simulink model "PV_MEV"  (R2025a)
settings: Solver=VariableStepAuto  StartTime=0.0  StopTime=10.0  RelTol=1e-3
InitFcn:
  | init_paras
values from neighbouring files (symbols this model uses):
  C_PFC = 2600e-6    (= 0.0026)    [init_paras.m]
  chg_ctrl_par = [Icc Vcv V_hys T_hys Kp_v_chg Ki_v_chg Kp_i_chg Ki_i_chg Ts_chg D_max_chg t_chg_on k_chg]    [init_paras.m]
  chg_ev = [0 Icc]    [init_paras.m]
  chg_par = [L_chg Voc Rint Ts_chg I_SIGN t_chg_on]    [init_paras.m]
  D = struct('X', {}, 'ti', {}, 'ia', {}, 'tc', {}, 'irms', {}, 'thd', {}, 'trip', {}, 'ttrip', {})    [make_waveform_figs.m]    (also in run_benchmark.m = get_sig('D'))
  det_ema_alpha = 0.1    [init_paras.m]
  det_force = 0    [init_paras.m]
  det_hyst = 0.6    [init_paras.m]
  det_persist = 2    [init_paras.m]
  det_src = 0    [init_paras.m]
  det_t_arm = 0.58    [init_paras.m]
  det_thr = [0.5 0.5 0.5 0.5 0.5]    [init_paras.m]
  det_variant_onehot = double(det_vlist == VARIANT_NAME)    [init_paras.m]
  ENABLE_HIL = 0    [init_paras.m]
  ENABLE_HIL_DET = 0    [init_paras.m]
  ENABLE_HIL_EST = 0    [init_paras.m]
  estimation_src = cfg_row.estimation_src    [init_paras.m]
  Fnom = 50    [init_paras.m]
  Fr_I = Fnom*2    (= 100)    [init_paras.m]
  grid_df = 0    [init_paras.m]
  grid_h5 = 0    [init_paras.m]
  grid_h7 = 0    [init_paras.m]
  grid_var_t0 = 0.7    [init_paras.m]
  hgq_fusion_alpha = [0.6704476522845647 0.7221651725151749 0.6446423751787858 0.41926421682656173]    [init_paras.m]
  hgq_min_ratio = single(0)    [init_paras.m]
  inj_channel = INJ.channel    [init_paras.m]
  inj_dwell = INJ.dwell    [init_paras.m]
  inj_shape = INJ.shape    [init_paras.m]
  inj_t_on = INJ.t_on    [init_paras.m]
  Ki_V = 80    [init_paras.m]
  Kp_I = 0.06    [init_paras.m]
  Kp_V = 0.25    [init_paras.m]
  Kr_I = 2.5    [init_paras.m]
  L_PFC = 600e-6    (= 0.0006)    [init_paras.m]
  Limit_V = 100    [init_paras.m]
  mit_t_ramp = 0.06    [init_paras.m]
  mitigation_mask = 0    [init_paras.m]
  mm_10cycle_points = mm_points_per_cycle * 10    (= 800)    [init_paras.m]
  mm_fund_freq = 50    [init_paras.m]
  mm_points_per_cycle = 80    [init_paras.m]
  R_bleed = 100e3    (= 100000)    [init_paras.m]
  R_pre = Ro*2    (= 44.44)    [init_paras.m]
  res_par = double(RES.par(:)'); end    [init_paras.m]
  RL_PFC = 20e-3    (= 0.02)    [init_paras.m]
  Ro = 22.22    [init_paras.m]
  t_pre_off = 0.30    (= 0.3)    [init_paras.m]
  Ts_chg = 10e-6    (= 1e-05)    [init_paras.m]
  Ts_Control = 1/Fc    [init_paras.m]
  Ts_Power = 50e-9    (= 5e-08)    [init_paras.m]    (also in run_benchmark.m = evalin('base','Ts_Power'))
  use_d_predict = cfg_row.use_d_predict    [init_paras.m]
  use_detector = 0    [init_paras.m]
  use_harmonic = cfg_row.use_harmonic    [init_paras.m]
  use_p_predict = cfg_row.use_p_predict    [init_paras.m]
  Vnom_ac = 240    [init_paras.m]
  vref_ev = [0 0]    [init_paras.m]
undefined symbols (not defined in the file or in its folder): D1, Delta, DiscIntNeverNeededParam
libraries: spsSeriesRLCBranchLib x17, spsMeanLib x16, MyLibrary x12, spsCurrentMeasurementLib x9, spsFourierLib x8, spsTHDLib x8, spsVoltageMeasurementLib x8, spsDiodeLib x7, simulink x7, pycoexlib x5, instrumentlib x4, spsPWMGeneratorDCDCLib x4
(part 4 of 7)

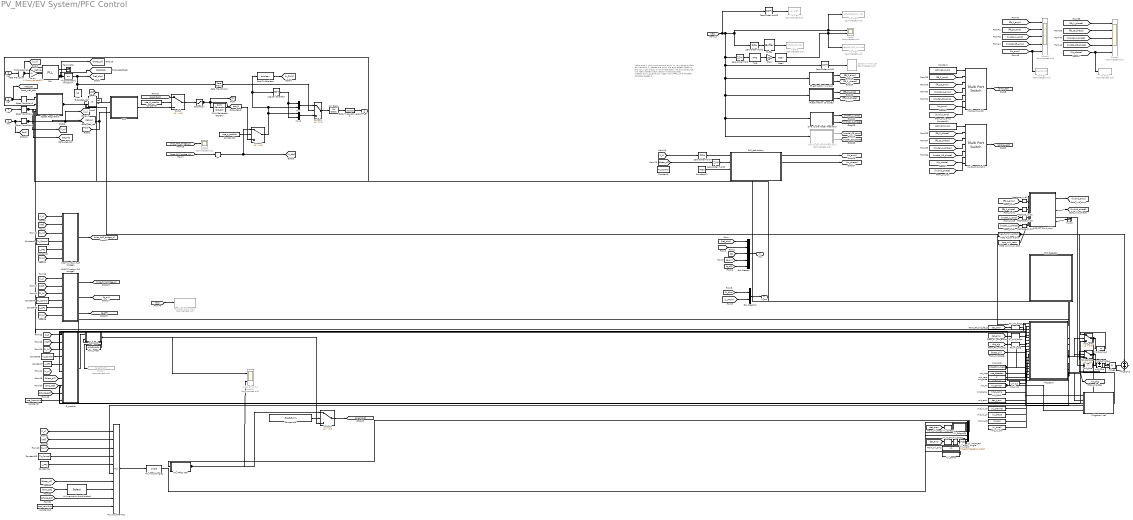
== system PV_MEV/EV System/PFC Control ==
  note: Make sure
      | 1. onnxruntime and onnx in your base python enviroment.
      | 2. reload the onnx file and refresh them in the onnx call block.
      | or comment them like this
      | otherwise will lead matlab crash
      |
      | (bash)
      | conda activate matlab_onnx_py310
      | pip install onnx==1.14.0
      |
      | (matlab console)
      | target = "/home/changhong/anaconda3/envs/matlab_onnx_py310/bin/python";
      | pe = pyenv
      | pyenv("Version", target)
  Vref : Inport
  Vdc : Inport  Port=2
  Vac : Inport  Port=3
  Iac : Inport  Port=4
  AbsI : Abs  SaturateOnIntegerOverflow=off
  AbsV : Abs  SaturateOnIntegerOverflow=off
  Buffer : Buffer  N=80  V=79  OutputFrames=off
  Bus Creator : BusCreator  Inputs=5
  Bus Creator1 : BusCreator  Inputs=2
  Cast To Boolean : DataTypeConversion  OutDataTypeStr=boolean  SaturateOnIntegerOverflow=off  RndMeth=Floor
  Constant : Constant  Value=estimation_src
  Constant{1..2,4,6,13} (5 alike) : Constant  Value=Ts_Control
  Constant10 : Constant  Value=use_p_predict
  Constant11 : Constant  Value=estimation_src
  Constant12 : Constant  Value=4000
  Constant{3,5,7,14} (4 alike) : Constant  Value=L_PFC
  Constant15 : Constant  Value=use_harmonic
  Constant16 : Constant  Value=ENABLE_HIL
  Constant8 : Constant  Value=use_harmonic
  Constant9 : Constant  Value=use_d_predict
  D_predict : MATLAB Function  TreatAsAtomicUnit=on
  Data Type Conversion2 : DataTypeConversion  OutDataTypeStr=double  SaturateOnIntegerOverflow=off  RndMeth=Floor
  EMI Detector : Subsystem
  Enabled Subsystem : Subsystem  Commented=on  TreatAsAtomicUnit=on
  Gain : Gain  Gain=100
  Goto17 : Goto  Commented=on  GotoTag=predict_D
  HGQ FFT-DL Hybrid : MATLAB Function  TreatAsAtomicUnit=on
  HGQ fusion alpha : Constant  Value=hgq_fusion_alpha(:)
  HGQ minimum ratio : Constant  Value=hgq_min_ratio
  HIL Harmonic Amplitudes1 : Selector  InputPortWidth=4  IndexOptions=Index vector (dialog)  Indices=[2 3 4]  OutputSizes=1
  HIL Input Frame1 : Mux  Inputs=10
  HIL Input Single1 : DataTypeConversion  OutDataTypeStr=single  SaturateOnIntegerOverflow=off  RndMeth=Floor
  HIL MPCC TCP : MATLAB Function  TreatAsAtomicUnit=on
  Half Cycle Model Prediction : Subsystem  Commented=on
  Logical Operator : Logic  Operator=NOT  AllPortsSameDT=off  OutDataTypeStr=float('double')
  MCP Function Half bridge1 : MATLAB Function  TreatAsAtomicUnit=on
  Mean : spsMeanLib/Mean  Freq=50  Vinit=0  Ts=1/4000
  Mitigation : MATLAB Function  TreatAsAtomicUnit=on
  Mitigation Iref : MATLAB Function  TreatAsAtomicUnit=on
  Multiport Switch : MultiPortSwitch  Inputs=6  SaturateOnIntegerOverflow=off  InputSameDT=off
  Multiport Switch1 : MultiPortSwitch  Inputs=6  SaturateOnIntegerOverflow=off  InputSameDT=off
  Mux : Mux  Inputs=2
  Mux2 : Mux  Inputs=2
  On Delay : spsOnDelayLib/On Delay  DelayType=On delay  delay=DT_PFC  ic=0  Ts=Ts_Power
  One  Cycle Model Prediction : Subsystem
  Original vs HIL Predict : Scope  Commented=on  NumInputPorts=2
      settings: DataLoggingSaveFormat=Array
  PLL : spsPLLLib/PLL  Fmin=0.9*Fnom  Par_Init=[0, Fnom]  ParK=[180, 3200, 1]  TcD=1e-4  MaxRateChangeFreq=12  FilterCutOffFreq=25  Ts=Ts_Control  AGC=on
  PR2 : Subsystem  mask(Current Regulator (Pr)){Kp=Kp_I, Kr=Kr_I, Fr=Fr_I}
      mask prompts: Kp "Proportional gain"; Kr "Resonant gain"; Fr "Resonant frequency (Hz)"
      mask help: This block implements a currentregulator using a PR controller.
      mask Display: disp('Current Regulator\n PR');
  PWM Generator (DC-DC) : spsPWMGeneratorDCDCLib/PWM Generator (DC-DC)  Fsw=Fsw  Ts=Ts_Power
  Prod1 : Product
  RLS_estimation : MATLAB Function  TreatAsAtomicUnit=on
  RT : RateTransition  OutPortSampleTime=5e-08
  RT_mit_amps : RateTransition  OutPortSampleTime=Ts_Control
  RT_mit_chg : RateTransition  OutPortSampleTime=Ts_Control
  RT_mit_flags : RateTransition  OutPortSampleTime=Ts_Control
  Rate Transition{,3..5} (4 alike) : RateTransition  OutPortSampleTime=Ts_Control
  Rate Transition2 : RateTransition  OutPortSampleTime=Ts_Power
  Reshape_hyb{1..4} (4 alike) : Reshape  OutputDimensionality=Column vector (2-D)
  Saturation : Saturate  UpperLimit=1  LowerLimit=0
  Scope : Scope  Commented=on  NumInputPorts=2
      settings: ActiveDisplayYMinimum=-211.219  ActiveDisplayYMaximum=223.7073  DataLoggingVariableName=ScopeData4  DataLoggingSaveFormat=Array
  Scope1 : Scope  Commented=on  NumInputPorts=5
      settings: ActiveDisplayYMinimum=-19.4864  ActiveDisplayYMaximum=175.3777  DataLoggingVariableName=ScopeData5  DataLoggingSaveFormat=Array
  Scope2 : Scope  Commented=on
      settings: DataLoggingVariableName=ScopeData9  DataLoggingSaveFormat=Array
  Scope3 : Scope  Commented=on  NumInputPorts=5
      settings: ActiveDisplayYMinimum=-3.927  ActiveDisplayYMaximum=3.927  DataLoggingVariableName=ScopeData6  DataLoggingSaveFormat=Array
  Spectrum Analyzer : SpectrumAnalyzer  Commented=on  WindowPosition=[-2559.000000,62.000000,1707.000000,996.000000,]  ScopeFrameLocation=window  SampleRateSource=Property  SampleRate=8000  PlotAsTwoSidedSpectrum=off  WindowInvariantSamplesPerUpdate=on  FrequencySpan=Start and stop frequencies  StartFrequency=0  StopFrequency=2000  YLimits=[-21.57310057,75.63654601]  ColorLimits=[-42.4528 59.157]
  Speed Regulator2 : Subsystem  DialogController=POWERSYS.PowerSysDialog  mask(Voltage Regulator){Kp=Kp_V, Ki=Ki_V, Limit_wreg=Limit_V, Init=0, Ts=Ts_Control}
      mask prompts: Kp "Proportional gain (Kp):"; Ki "Integral gain (Ki):"; Limit_wreg "Output limits"; Init "Output initial value:"; Ts "Sample time:"
      mask help: This block implements a voltage regulator using an ant-windup PI controller.
      mask Display: disp('Voltage\nRegulator');
  Switch : Switch  Criteria=u2 > Threshold  Threshold=0.5  SaturateOnIntegerOverflow=off  InputSameDT=off
  Switch1 : Switch  SaturateOnIntegerOverflow=off  InputSameDT=off
  Switch2 : Switch  Criteria=u2 > Threshold  Threshold=0.5  SaturateOnIntegerOverflow=off  InputSameDT=off
  Switch3 : Switch  Criteria=u2 > Threshold  Threshold=0.5  SaturateOnIntegerOverflow=off  InputSameDT=off
  THD : spsTHDLib/THD  Freq=50  Ts=1/4000
  T_hyb : Terminator
  Terminator : Terminator
  To File : ToFile  Commented=on  Filename=MPCC_IAC.mat  SaveFormat=Timeseries
  To File1 : ToFile  Commented=on  Filename=rls_phase.mat  SaveFormat=Timeseries
  To File2 : ToFile  Commented=on  Filename=rls_amp.mat  SaveFormat=Timeseries
  To File3 : ToFile  Commented=on  Filename=Iac.mat  SaveFormat=Timeseries
  To File4 : ToFile  Commented=on  Filename=results/Iac_ori.mat  SaveFormat=Timeseries
  To File5 : ToFile  Commented=on  Filename=results/THD_ori.mat  SaveFormat=Timeseries
  Trigonometric Function7 : Trigonometry
  UMPC Function Full bridge1 : MATLAB Function  TreatAsAtomicUnit=on
  Zero-Order Hold{,1,3..5} (5 alike) : ZeroOrderHold  SampleTime=1/4000
  Zero-Order Hold2 : ZeroOrderHold  SampleTime=1/8000
  fft estimation 1 cycle2 : Subsystem
  fft estimation 10 cycle2 : Subsystem
  hil_amp3 : Selector  InputPortWidth=5  IndexOptions=Index vector (dialog)  Indices=3  OutputSizes=1
  hil_amp3_single : DataTypeConversion  OutDataTypeStr=single  SaturateOnIntegerOverflow=off  RndMeth=Floor
  hil_flagword : MATLAB Function  TreatAsAtomicUnit=on
  hil_mask : Constant  Value=single(mitigation_mask)
  hil_mpcc_ext : Mux  Inputs=5
  hil_rt_amp : RateTransition  OutPortSampleTime=Ts_Control
  hil_rt_flags : RateTransition  OutPortSampleTime=Ts_Control
  hil_tramp : Constant  Value=single(mit_t_ramp)
  hold_amp : Switch  Criteria=u2 > Threshold  Threshold=0.5  SaturateOnIntegerOverflow=off  InputSameDT=off
  hold_amp_z : UnitDelay  SampleTime=Ts_Control  HasFrameUpgradeWarning=on
  hold_mask : FromWorkspace  VariableName=HOLDMASK  SampleTime=Ts_Control  Interpolate=off  OutputAfterFinalValue=Holding final value
  hold_phase : Switch  Criteria=u2 > Threshold  Threshold=0.5  SaturateOnIntegerOverflow=off  InputSameDT=off
  hold_phase_z : UnitDelay  SampleTime=Ts_Control  HasFrameUpgradeWarning=on
  mit_1ma : Sum  Inputs=+-
  mit_Ts : Constant  Value=Ts_Control
  mit_alpha : Sum
  mit_clock : DigitalClock  SampleTime=Ts_Control
  mit_force : Constant  Value=det_force
  mit_ga : Product
  mit_ilim0 : Constant  Value=Limit_V
  mit_inj_ch : Constant  Value=inj_channel
  mit_inj_dw : Constant  Value=inj_dwell
  mit_inj_sh : Constant  Value=inj_shape
  mit_inj_t0 : Constant  Value=inj_t_on
  mit_mask : Constant  Value=mitigation_mask
  mit_one : Constant
  mit_tarm : Constant  Value=det_t_arm
  mit_tramp : Constant  Value=mit_t_ramp
  mit_use : Constant  Value=use_detector
  mit_zero : Constant  Value=0
  tick_hold : MATLAB Function  TreatAsAtomicUnit=on
  to-pu : Gain  Gain=1/(Vnom_ac*sqrt(2))
  g1_g2 : Outport  PortDimensions=2
  Sig : Outport  Port=2
  u_swt : Outport  Port=3
  tag scope: Vref_det=global, det_D=global, det_Iac=global, det_Iref=global, det_Vac=global, det_Vdc=global, det_theta=global, mit_dbg=global
  wires:
  Mux/1 -> Switch1/1
  Iac/1 -> [Iac], Rate Transition5/1
  Speed Regulator2/1(Out) -> [det_Iref], Mitigation Iref/1(Iref)
  Rate Transition2/1 -> Switch1/2
  Data Type Conversion2/1 -> g1_g2/1
  PLL/2 -> [theta_pll], Trigonometric Function7/1, [det_theta]
  Saturation/1 -> PWM Generator (DC-DC)/1, [D], [det_D]
  to-pu/1 -> PLL/1
  Rate Transition/1 -> [V_in], to-pu/1, [det_Vac]
  Bus Creator1/1 -> u_swt/1
  AbsI/1 -> PR2/2(Iac), [Iac_abs]
  Trigonometric Function7/1 -> AbsV/1, Rate Transition2/1, [Iref_obs]
  [D] -> Bus Creator/3  "D"
  Rate Transition3/1 -> Speed Regulator2/1(Vref)
  Switch1/1 -> On Delay/1
  Rate Transition4/1 -> [det_Vdc], [V_o], Mitigation/3(Vdc)
  [u_obs] -> Bus Creator1/1  "u_obs"
  Mux2/1 -> Switch1/3
  Vdc/1 -> Rate Transition4/1
  [mcp_full_bridge_o] -> RT/1
  [Iref_obs] -> Bus Creator/1  "Iref_obs"
  RT/1 -> Switch2/1, [u_obs]
  Cast To Boolean/1 -> [u_PWM]
  PWM Generator (DC-DC)/1 -> Switch2/3
  Vac/1 -> Rate Transition/1
  Prod1/1 -> [Iref], PR2/1(Iref)
  Bus Creator/1 -> Sig/1
  Rate Transition5/1 -> [i_L], AbsI/1, [det_Iac]
  PLL/1 -> Terminator/1
  AbsV/1 -> Prod1/1
  [Iac_abs] -> Bus Creator/2  "Iac_abc"
  Switch2/1 -> Logical Operator/1, Cast To Boolean/1, Mux/2, Mux2/1
  Vref/1 -> Rate Transition3/1, [Vref_det]
  On Delay/1 -> Data Type Conversion2/1
  [u_PWM] -> Bus Creator1/2  "u_PWM"
  [Iac] -> Zero-Order Hold3/1, Half Cycle Model Prediction/1(u), One  Cycle Model Prediction/1(u), fft estimation 10 cycle2/1(u), fft estimation 1 cycle2/1(u), Zero-Order Hold2/1, Zero-Order Hold/1, Zero-Order Hold1/1, To File4/1, Scope/1  "Iac"
  Buffer/1 -> To File/1
  Gain/1 -> Mean/1
  Zero-Order Hold/1 -> THD/1
  Mean/1 -> To File5/1, Scope/2
  Zero-Order Hold2/1 -> Spectrum Analyzer/1
  THD/1 -> Gain/1
  Zero-Order Hold1/1 -> Buffer/1
  [i_L] -> MCP Function Half bridge1/1(i_L)
  [Iref] -> MCP Function Half bridge1/2(i_ref)
  [V_in] -> MCP Function Half bridge1/3(V_in)
  Constant2/1 -> MCP Function Half bridge1/4(Ts)
  Constant3/1 -> MCP Function Half bridge1/5(L_in)
  [V_o] -> MCP Function Half bridge1/6(V_o)
  MCP Function Half bridge1/1(y) -> [mcp_half_bridge_o]
  [i_L] -> UMPC Function Full bridge1/1(i_L)
  [Iref] -> UMPC Function Full bridge1/2(i_ref)
  [V_in] -> UMPC Function Full bridge1/3(V_in)
  Constant4/1 -> UMPC Function Full bridge1/4(Ts)
  Constant5/1 -> UMPC Function Full bridge1/5(L_in)
  [V_o] -> UMPC Function Full bridge1/6(V_o)
  UMPC Function Full bridge1/1(y) -> [mcp_full_bridge_o]
  UMPC Function Full bridge1/2(g_on) -> [g_on]
  UMPC Function Full bridge1/3(g_off) -> [g_off]
  [g_on] -> Bus Creator/4  "g_on"
  [g_off] -> Bus Creator/5  "g_off"
  [theta_pll] -> Zero-Order Hold5/1
  [Iref] -> D_predict/2(i_ref)
  Constant6/1 -> D_predict/4(Ts)
  Constant7/1 -> D_predict/5(L_in)
  Constant8/1 -> D_predict/10(use_harmonic)
  [theta_pll] -> D_predict/7(theta_pll)
  [mcp_half_bridge_o] -> Scope2/1
  Constant9/1 -> Switch/2
  [predict_D] -> Switch/1
  PR2/1(D) -> Switch/3
  Switch/1 -> Saturation/1
  Constant10/1 -> Switch2/2
  Logical Operator/1 -> Mux2/2, Mux/1
  Constant/1 -> Multiport Switch/1
  fft estimation 1 cycle2/1(amp) -> [fft_1_amp]
  fft estimation 1 cycle2/2(phase) -> [fft_1_phase]
  fft estimation 10 cycle2/1(amp) -> [fft_10_amp]
  fft estimation 10 cycle2/2(phase) -> [fft_10_phase]
  One  Cycle Model Prediction/1(amplitude) -> [model_1_amp]
  One  Cycle Model Prediction/2(phase) -> [model_1_phase]
  Half Cycle Model Prediction/1(amplitude) -> [model_05_amp]  "amp_est"
  Half Cycle Model Prediction/2(phase) -> [model_05_phase]  "hase_est"
  Multiport Switch/1 -> [amp_est]
  RLS_estimation/1(amp_est) -> [rls_amp]
  RLS_estimation/2(phase_est) -> [rls_phase]
  [fft_1_amp] -> Multiport Switch/2
  [fft_10_amp] -> Multiport Switch/3
  [model_1_amp] -> Multiport Switch/4
  [model_05_amp] -> Multiport Switch/5
  [rls_amp] -> Multiport Switch/6
  [rls_phase] -> Multiport Switch1/6
  [model_05_phase] -> Multiport Switch1/5
  [model_1_phase] -> Multiport Switch1/4
  [fft_10_phase] -> Multiport Switch1/3
  [fft_1_phase] -> Multiport Switch1/2
  Multiport Switch1/1 -> [phase_est]
  Constant11/1 -> Multiport Switch1/1
  [fft_1_amp] -> Scope1/1
  [fft_10_amp] -> Scope1/2
  [model_1_amp] -> Scope1/3
  [model_05_amp] -> Scope1/4
  [rls_amp] -> To File2/1, Scope1/5
  [fft_1_phase] -> Scope3/1
  [fft_10_phase] -> Scope3/2
  [model_1_phase] -> Scope3/3
  [model_05_phase] -> Scope3/4
  [rls_phase] -> To File1/1, Scope3/5
  Zero-Order Hold3/1 -> To File3/1
  [i_L] -> Zero-Order Hold4/1
  Constant12/1 -> RLS_estimation/3(Ts)
  Zero-Order Hold4/1 -> RLS_estimation/1(i_L)
  Zero-Order Hold5/1 -> RLS_estimation/2(theta_pll)
  [Iac] -> Enabled Subsystem/1(Iac)  "Iac"
  [amp_est] -> HIL Harmonic Amplitudes1/1
  [i_L] -> HIL Input Frame1/1
  [Iref] -> HIL Input Frame1/2
  [V_in] -> HIL Input Frame1/3
  Constant13/1 -> HIL Input Frame1/4
  Constant14/1 -> HIL Input Frame1/5
  [theta_pll] -> HIL Input Frame1/7
  HIL Harmonic Amplitudes1/1 -> HIL Input Frame1/8
  [phase_est] -> HIL Input Frame1/9
  Constant15/1 -> HIL Input Frame1/10
  HIL Input Frame1/1 -> HIL Input Single1/1
  Switch3/1 -> [predict_D]
  Constant16/1 -> Switch3/2
  [fft_1_amp] -> Reshape_hyb1/1
  Reshape_hyb1/1 -> HGQ FFT-DL Hybrid/1(fft_amplitude)
  [fft_1_phase] -> Reshape_hyb2/1
  Reshape_hyb2/1 -> HGQ FFT-DL Hybrid/2(fft_phase)
  [model_1_amp] -> Reshape_hyb3/1
  Reshape_hyb3/1 -> HGQ FFT-DL Hybrid/3(dl_amplitude)
  [model_1_phase] -> Reshape_hyb4/1
  Reshape_hyb4/1 -> HGQ FFT-DL Hybrid/4(dl_phase)
  HGQ minimum ratio/1 -> HGQ FFT-DL Hybrid/6(minimum_ratio)
  HGQ FFT-DL Hybrid/1(amplitude_out) -> [hybrid_amp]
  HGQ FFT-DL Hybrid/2(phase_out) -> [hybrid_phase]
  HGQ FFT-DL Hybrid/3(dl_accepted) -> T_hyb/1
  [hybrid_amp] -> Multiport Switch/7
  [hybrid_phase] -> Multiport Switch1/7
  [det_chan] -> RT_mit_flags/1
  RT_mit_flags/1 -> Mitigation/1(flags)
  [det_amp] -> RT_mit_amps/1
  RT_mit_amps/1 -> Mitigation/2(amps)
  [chg_sig] -> RT_mit_chg/1
  RT_mit_chg/1 -> Mitigation/8(chg)
  mit_mask/1 -> Mitigation/9(mask), Mitigation Iref/3(mask)
  mit_use/1 -> Mitigation/10(use_det)
  mit_force/1 -> Mitigation/11(force)
  mit_Ts/1 -> Mitigation/12(Ts), Mitigation Iref/4(Ts)
  mit_tramp/1 -> Mitigation/13(t_ramp)
  Mitigation/1(Vdc_fb) -> Speed Regulator2/2(Vmeas)
  [i_L] -> Mitigation/6(iL)
  Mitigation/4(iL_out) -> D_predict/1(i_L)
  [V_in] -> Mitigation/4(Vac)
  Mitigation/3(Vin_out) -> D_predict/3(V_in)
  [theta_pll] -> Mitigation/5(th)
  [amp_est] -> hold_amp/3
  hold_amp/1 -> D_predict/8(amp_est), hold_amp_z/1
  hold_amp_z/1 -> hold_amp/1
  Mitigation/5(hold) -> hold_amp/2, hold_phase/2
  [phase_est] -> hold_phase/3
  hold_phase/1 -> D_predict/9(phase_est), hold_phase_z/1
  hold_phase_z/1 -> hold_phase/1
  mit_one/1 -> mit_1ma/1
  HGQ fusion alpha/1 -> mit_1ma/2, mit_alpha/1
  mit_1ma/1 -> mit_ga/1
  Mitigation/6(g_alpha) -> mit_ga/2
  mit_ga/1 -> mit_alpha/2
  mit_alpha/1 -> HGQ FFT-DL Hybrid/5(alpha)
  Mitigation/7(dbg) -> [mit_dbg], Mitigation Iref/2(dbg)
  mit_zero/1 -> Mitigation/7(Iref)
  Mitigation Iref/1(Iref_out) -> Prod1/2
  mit_clock/1 -> Mitigation/14(tnow)
  mit_tarm/1 -> Mitigation/15(t_arm)
  HIL Input Single1/1 -> hil_mpcc_ext/1
  [det_chan] -> hil_rt_flags/1
  hil_rt_flags/1 -> hil_flagword/1(c)
  hil_flagword/1(w) -> hil_mpcc_ext/2
  [det_amp] -> hil_rt_amp/1
  hil_rt_amp/1 -> hil_amp3/1
  hil_amp3/1 -> hil_amp3_single/1
  hil_amp3_single/1 -> hil_mpcc_ext/3
  hil_mask/1 -> hil_mpcc_ext/4
  hil_tramp/1 -> hil_mpcc_ext/5
  hil_mpcc_ext/1 -> HIL MPCC TCP/1(x)
  HIL MPCC TCP/1(y) -> Original vs HIL Predict/2, Switch3/1
  mit_inj_ch/1 -> Mitigation/16(inj_ch)
  mit_inj_sh/1 -> Mitigation/17(inj_sh)
  mit_inj_t0/1 -> Mitigation/18(inj_t0)
  mit_inj_dw/1 -> Mitigation/19(inj_dw)
  D_predict/1(D) -> tick_hold/1(D)
  hold_mask/1 -> tick_hold/2(hold)
  tick_hold/1(Dout) -> Switch3/3, Original vs HIL Predict/1, Goto17/1
  mit_ilim0/1 -> Mitigation/20(Ilim0)
  Mitigation/8(Ilim) -> Speed Regulator2/3(Ilim)
  Mitigation/9(Vo_ctl) -> D_predict/6(V_o), HIL Input Frame1/6

== system PV_MEV/EV System/Subsystem ==

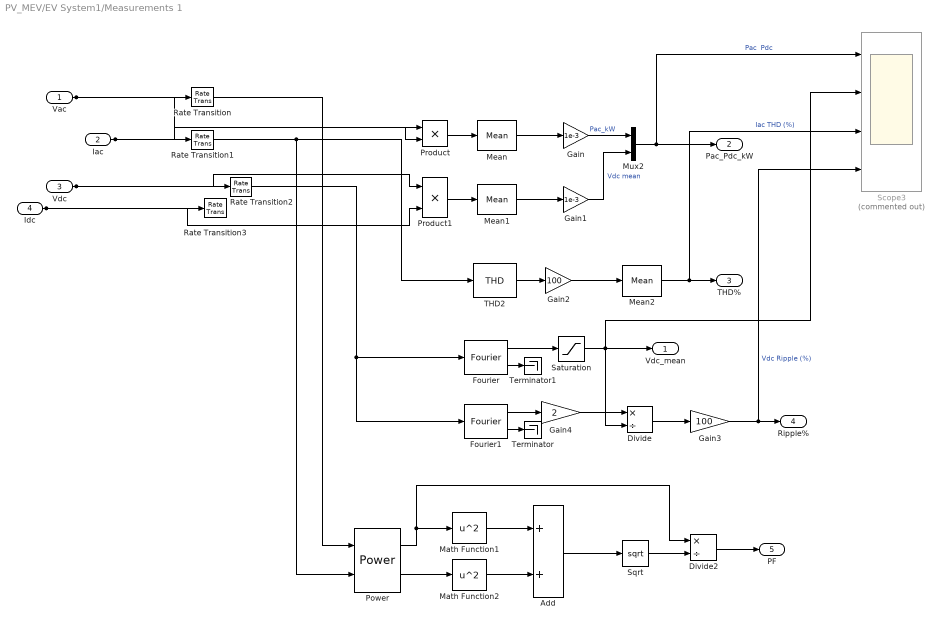
== system PV_MEV/EV System1/Measurements 1 ==
  Vac : Inport
  Iac : Inport  Port=2
  Vdc : Inport  Port=3
  Idc : Inport  Port=4
  Add : Sum
  Divide : Product  Inputs=*/
  Divide2 : Product  Inputs=*/
  Fourier : spsFourierLib/Fourier  Freq=Fnom  n=0  InInit=[0, 0]  Ts=Ts_Control
  Fourier1 : spsFourierLib/Fourier  Freq=Fnom  n=2  InInit=[0, 0]  Ts=Ts_Control
  Gain : Gain  Gain=1e-3
  Gain1 : Gain  Gain=1e-3
  Gain2 : Gain  Gain=100
  Gain3 : Gain  Gain=100
  Gain4 : Gain  Gain=2
  Math Function1 : Math  Operator=square
  Math Function2 : Math  Operator=square
  Mean : spsMeanLib/Mean  Freq=Fnom  Vinit=0  Ts=Ts_Power
  Mean1 : spsMeanLib/Mean  Freq=Fnom  Vinit=0  Ts=Ts_Power
  Mean2 : spsMeanLib/Mean  Freq=Fnom  Vinit=0  Ts=Ts_Control
  Mux2 : Mux  Inputs=2
  Power : spsPowerLib/Power  Freq=Fnom  Vinit=[1, 0]  Iinit=[1, 0]  Ts=Ts_Control
  Product : Product
  Product1 : Product
  Rate Transition{,1..3} (4 alike) : RateTransition  OutPortSampleTime=Ts_Control
  Saturation : Saturate  UpperLimit=inf  LowerLimit=eps
  Scope3 : Scope  Commented=on  NumInputPorts=4
      settings: DataLoggingSaveFormat=Array
  Sqrt : Sqrt
  THD2 : spsTHDLib/THD  Freq=Fnom  Ts=Ts_Control
  Terminator : Terminator
  Terminator1 : Terminator
  Vdc_mean : Outport
  Pac_Pdc_kW : Outport  Port=2
  THD% : Outport  Port=3
  Ripple% : Outport  Port=4
  PF : Outport  Port=5
  wires:
  Rate Transition2/1 -> Fourier1/1, Fourier/1
  Vac/1 -> Rate Transition/1, Product/1
  Rate Transition/1 -> Power/1
  Idc/1 -> Rate Transition3/1, Product1/2
  Vdc/1 -> Rate Transition2/1, Product1/1
  Rate Transition1/1 -> Power/2, THD2/1
  Divide2/1 -> PF/1
  Sqrt/1 -> Divide2/2
  Add/1 -> Sqrt/1
  Math Function2/1 -> Add/2
  Math Function1/1 -> Add/1
  Power/2 -> Math Function2/1
  Power/1 -> Divide2/1, Math Function1/1
  Gain3/1 -> Ripple%/1, Scope3/4  "Vdc Ripple (%)"
  Fourier1/2 -> Terminator/1
  Gain4/1 -> Divide/1
  Fourier1/1 -> Gain4/1
  Divide/1 -> Gain3/1
  Saturation/1 -> Divide/2, Vdc_mean/1, Scope3/2
  Fourier/1 -> Saturation/1
  Fourier/2 -> Terminator1/1
  Mean2/1 -> THD%/1, Scope3/3  "Iac THD (%)"
  Gain2/1 -> Mean2/1
  Mux2/1 -> Pac_Pdc_kW/1, Scope3/1  "Pac  Pdc"
  Iac/1 -> Rate Transition1/1, Product/2
  Mean1/1 -> Gain1/1
  THD2/1 -> Gain2/1
  Gain/1 -> Mux2/1  "Pac_kW"
  Product/1 -> Mean/1
  Mean/1 -> Gain/1
  Product1/1 -> Mean1/1
  Gain1/1 -> Mux2/2  "Vdc mean"

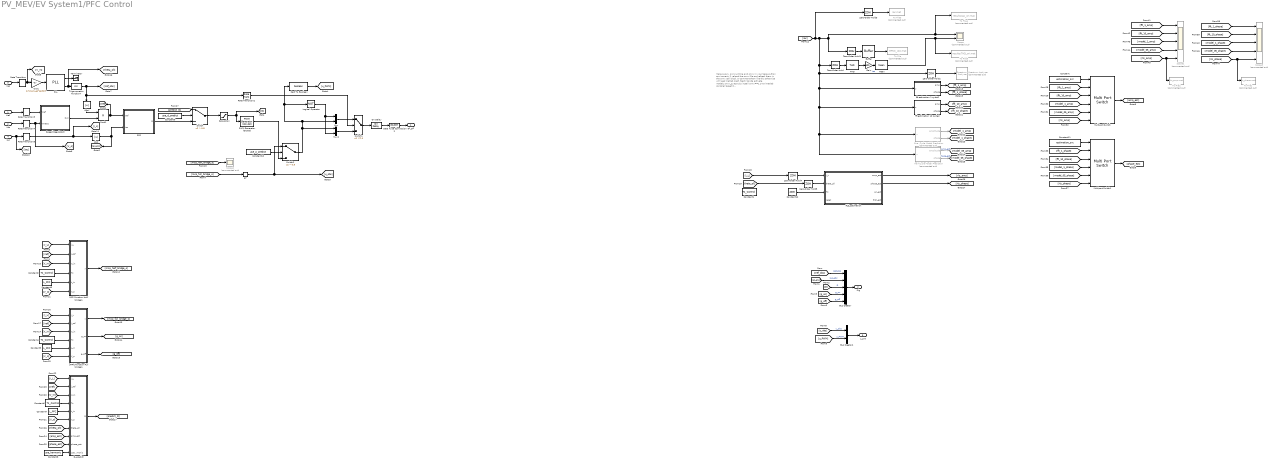
== system PV_MEV/EV System1/PFC Control ==
  note: Make sure
      | 1. onnxruntime and onnx in your base python enviroment.
      | 2. reload the onnx file and refresh them in the onnx call block.
      | or comment them like this
      | otherwise will lead matlab crash
      |
      | (bash)
      | conda activate matlab_onnx_py310
      | pip install onnx==1.14.0
      |
      | (matlab console)
      | target = "/home/changhong/anaconda3/envs/matlab_onnx_py310/bin/python";
      | pe = pyenv
      | pyenv("Version", target)
  Vref : Inport
  Vdc : Inport  Port=2
  Vac : Inport  Port=3
  Iac : Inport  Port=4
  AbsI : Abs  SaturateOnIntegerOverflow=off
  AbsV : Abs  SaturateOnIntegerOverflow=off
  Buffer : Buffer  N=80  V=79  OutputFrames=off
  Bus Creator : BusCreator  Inputs=5
  Bus Creator1 : BusCreator  Inputs=2
  Cast To Boolean : DataTypeConversion  OutDataTypeStr=boolean  SaturateOnIntegerOverflow=off  RndMeth=Floor
  Constant : Constant  Value=estimation_src
  Constant{1..2,4,6} (4 alike) : Constant  Value=Ts_Control
  Constant10 : Constant  Value=use_p_predict
  Constant11 : Constant  Value=estimation_src
  Constant12 : Constant  Value=4000
  Constant3 : Constant  Value=L_PFC
  Constant5 : Constant  Value=L_PFC
  Constant7 : Constant  Value=L_PFC
  Constant8 : Constant  Value=use_harmonic
  Constant9 : Constant  Value=use_d_predict
  D_predict : MATLAB Function  TreatAsAtomicUnit=on
  Data Type Conversion2 : DataTypeConversion  OutDataTypeStr=double  SaturateOnIntegerOverflow=off  RndMeth=Floor
  Gain : Gain  Gain=100
  Half Cycle Model Prediction : Subsystem  Commented=on
  Logical Operator : Logic  Operator=NOT  AllPortsSameDT=off  OutDataTypeStr=float('double')
  MCP Function Half bridge1 : MATLAB Function  TreatAsAtomicUnit=on
  Mean : spsMeanLib/Mean  Freq=50  Vinit=0  Ts=1/4000
  Multiport Switch : MultiPortSwitch  Inputs=5  SaturateOnIntegerOverflow=off  InputSameDT=off
  Multiport Switch1 : MultiPortSwitch  Inputs=5  SaturateOnIntegerOverflow=off  InputSameDT=off
  Mux : Mux  Inputs=2
  Mux2 : Mux  Inputs=2
  On Delay : spsOnDelayLib/On Delay  DelayType=On delay  delay=DT_PFC  ic=0  Ts=Ts_Power
  One  Cycle Model Prediction : Subsystem  Commented=on
  PLL : spsPLLLib/PLL  Fmin=0.9*Fnom  Par_Init=[0, Fnom]  ParK=[180, 3200, 1]  TcD=1e-4  MaxRateChangeFreq=12  FilterCutOffFreq=25  Ts=Ts_Control  AGC=on
  PR2 : Subsystem  mask(Current Regulator (Pr)){Kp=Kp_I, Kr=Kr_I, Fr=Fr_I}
      mask prompts: Kp "Proportional gain"; Kr "Resonant gain"; Fr "Resonant frequency (Hz)"
      mask help: This block implements a currentregulator using a PR controller.
      mask Display: disp('Current Regulator\n PR');
  PWM Generator (DC-DC) : spsPWMGeneratorDCDCLib/PWM Generator (DC-DC)  Fsw=Fsw  Ts=Ts_Power
  Prod1 : Product
  RLS_estimation : MATLAB Function  TreatAsAtomicUnit=on
  RT : RateTransition  OutPortSampleTime=5e-08
  Rate Transition{,3..5} (4 alike) : RateTransition  OutPortSampleTime=Ts_Control
  Rate Transition2 : RateTransition  OutPortSampleTime=Ts_Power
  Saturation : Saturate  UpperLimit=1  LowerLimit=0
  Scope : Scope  Commented=on  NumInputPorts=2
      settings: ActiveDisplayYMinimum=-211.219  ActiveDisplayYMaximum=223.7073  DataLoggingVariableName=ScopeData4  DataLoggingSaveFormat=Array
  Scope1 : Scope  Commented=on  NumInputPorts=5
      settings: ActiveDisplayYMinimum=-19.4864  ActiveDisplayYMaximum=175.3777  DataLoggingVariableName=ScopeData5  DataLoggingSaveFormat=Array
  Scope2 : Scope  Commented=on
      settings: DataLoggingVariableName=ScopeData9  DataLoggingSaveFormat=Array
  Scope3 : Scope  Commented=on  NumInputPorts=5
      settings: ActiveDisplayYMinimum=-3.927  ActiveDisplayYMaximum=3.927  DataLoggingVariableName=ScopeData6  DataLoggingSaveFormat=Array
  Spectrum Analyzer : SpectrumAnalyzer  Commented=on  WindowPosition=[-2559.000000,62.000000,1707.000000,996.000000,]  ScopeFrameLocation=window  SampleRateSource=Property  SampleRate=8000  PlotAsTwoSidedSpectrum=off  WindowInvariantSamplesPerUpdate=on  FrequencySpan=Start and stop frequencies  StartFrequency=0  StopFrequency=2000  YLimits=[-21.57310057,75.63654601]  ColorLimits=[-42.4528 59.157]
  Speed Regulator2 : Subsystem  DialogController=POWERSYS.PowerSysDialog  mask(Voltage Regulator){Kp=Kp_V, Ki=Ki_V, Limit_wreg=Limit_V, Init=0, Ts=Ts_Control}
      mask prompts: Kp "Proportional gain (Kp):"; Ki "Integral gain (Ki):"; Limit_wreg "Output limits"; Init "Output initial value:"; Ts "Sample time:"
      mask help: This block implements a voltage regulator using an ant-windup PI controller.
      mask Display: disp('Voltage\nRegulator');
  Switch : Switch  Criteria=u2 > Threshold  Threshold=0.5  SaturateOnIntegerOverflow=off  InputSameDT=off
  Switch1 : Switch  SaturateOnIntegerOverflow=off  InputSameDT=off
  Switch2 : Switch  Criteria=u2 > Threshold  Threshold=0.5  SaturateOnIntegerOverflow=off  InputSameDT=off
  THD : spsTHDLib/THD  Freq=50  Ts=1/4000
  Terminator : Terminator
  To File : ToFile  Commented=on  Filename=MPCC_IAC.mat  SaveFormat=Timeseries
  To File1 : ToFile  Commented=on  Filename=rls_phase.mat  SaveFormat=Timeseries
  To File2 : ToFile  Commented=on  Filename=rls_amp.mat  SaveFormat=Timeseries
  To File3 : ToFile  Commented=on  Filename=Iac.mat  SaveFormat=Timeseries
  To File4 : ToFile  Commented=on  Filename=results/Iac_ori.mat  SaveFormat=Timeseries
  To File5 : ToFile  Commented=on  Filename=results/THD_ori.mat  SaveFormat=Timeseries
  Trigonometric Function7 : Trigonometry
  UMPC Function Full bridge1 : MATLAB Function  TreatAsAtomicUnit=on
  Zero-Order Hold{,1,3..5} (5 alike) : ZeroOrderHold  SampleTime=1/4000
  Zero-Order Hold2 : ZeroOrderHold  SampleTime=1/8000
  fft estimation 1 cycle2 : Subsystem
  fft estimation 10 cycle2 : Subsystem
  to-pu : Gain  Gain=1/(Vnom_ac*sqrt(2))
  g1_g2 : Outport  PortDimensions=2
  Sig : Outport  Port=2
  u_swt : Outport  Port=3
  wires:
  Zero-Order Hold5/1 -> RLS_estimation/2(theta_pll)
  Zero-Order Hold4/1 -> RLS_estimation/1(i_L)
  Constant12/1 -> RLS_estimation/3(Ts)
  [i_L] -> Zero-Order Hold4/1
  Zero-Order Hold3/1 -> To File3/1
  [rls_phase] -> Scope3/5, To File1/1
  [model_05_phase] -> Scope3/4
  [model_1_phase] -> Scope3/3
  [fft_10_phase] -> Scope3/2
  [fft_1_phase] -> Scope3/1
  [rls_amp] -> Scope1/5, To File2/1
  [model_05_amp] -> Scope1/4
  [model_1_amp] -> Scope1/3
  [fft_10_amp] -> Scope1/2
  [fft_1_amp] -> Scope1/1
  Constant11/1 -> Multiport Switch1/1
  Multiport Switch1/1 -> [phase_est]
  [fft_1_phase] -> Multiport Switch1/2
  [fft_10_phase] -> Multiport Switch1/3
  [model_1_phase] -> Multiport Switch1/4
  [model_05_phase] -> Multiport Switch1/5
  [rls_phase] -> Multiport Switch1/6
  [rls_amp] -> Multiport Switch/6
  [model_05_amp] -> Multiport Switch/5
  [model_1_amp] -> Multiport Switch/4
  [fft_10_amp] -> Multiport Switch/3
  [fft_1_amp] -> Multiport Switch/2
  RLS_estimation/2(phase_est) -> [rls_phase]
  RLS_estimation/1(amp_est) -> [rls_amp]
  Multiport Switch/1 -> [amp_est]
  Half Cycle Model Prediction/2(phase) -> [model_05_phase]  "hase_est"
  Half Cycle Model Prediction/1(amplitude) -> [model_05_amp]  "amp_est"
  One  Cycle Model Prediction/2(phase) -> [model_1_phase]
  One  Cycle Model Prediction/1(amplitude) -> [model_1_amp]
  fft estimation 10 cycle2/2(phase) -> [fft_10_phase]
  fft estimation 10 cycle2/1(amp) -> [fft_10_amp]
  fft estimation 1 cycle2/2(phase) -> [fft_1_phase]
  fft estimation 1 cycle2/1(amp) -> [fft_1_amp]
  Constant/1 -> Multiport Switch/1
  Logical Operator/1 -> Mux/1, Mux2/2
  Constant10/1 -> Switch2/2
  Switch/1 -> Saturation/1
  PR2/1(D) -> Switch/3
  [predict_D] -> Switch/1
  Constant9/1 -> Switch/2
  [mcp_half_bridge_o] -> Scope2/1
  D_predict/1(D) -> [predict_D]
  [theta_pll] -> D_predict/7(theta_pll)
  Constant8/1 -> D_predict/10(use_harmonic)
  [phase_est] -> D_predict/9(phase_est)
  [amp_est] -> D_predict/8(amp_est)
  [V_o] -> D_predict/6(V_o)
  Constant7/1 -> D_predict/5(L_in)
  Constant6/1 -> D_predict/4(Ts)
  [V_in] -> D_predict/3(V_in)
  [Iref] -> D_predict/2(i_ref)
  [i_L] -> D_predict/1(i_L)
  [theta_pll] -> Zero-Order Hold5/1
  [g_off] -> Bus Creator/5  "g_off"
  [g_on] -> Bus Creator/4  "g_on"
  UMPC Function Full bridge1/3(g_off) -> [g_off]
  UMPC Function Full bridge1/2(g_on) -> [g_on]
  UMPC Function Full bridge1/1(y) -> [mcp_full_bridge_o]
  [V_o] -> UMPC Function Full bridge1/6(V_o)
  Constant5/1 -> UMPC Function Full bridge1/5(L_in)
  Constant4/1 -> UMPC Function Full bridge1/4(Ts)
  [V_in] -> UMPC Function Full bridge1/3(V_in)
  [Iref] -> UMPC Function Full bridge1/2(i_ref)
  [i_L] -> UMPC Function Full bridge1/1(i_L)
  MCP Function Half bridge1/1(y) -> [mcp_half_bridge_o]
  [V_o] -> MCP Function Half bridge1/6(V_o)
  Constant3/1 -> MCP Function Half bridge1/5(L_in)
  Constant2/1 -> MCP Function Half bridge1/4(Ts)
  [V_in] -> MCP Function Half bridge1/3(V_in)
  [Iref] -> MCP Function Half bridge1/2(i_ref)
  [i_L] -> MCP Function Half bridge1/1(i_L)
  Zero-Order Hold1/1 -> Buffer/1
  THD/1 -> Gain/1
  Zero-Order Hold2/1 -> Spectrum Analyzer/1
  Mean/1 -> Scope/2, To File5/1
  Zero-Order Hold/1 -> THD/1
  Gain/1 -> Mean/1
  Buffer/1 -> To File/1
  [Iac] -> Scope/1, To File4/1, Zero-Order Hold1/1, Zero-Order Hold/1, Zero-Order Hold2/1, fft estimation 1 cycle2/1(u), fft estimation 10 cycle2/1(u), One  Cycle Model Prediction/1(u), Half Cycle Model Prediction/1(u), Zero-Order Hold3/1  "Iac"
  [u_PWM] -> Bus Creator1/2  "u_PWM"
  On Delay/1 -> Data Type Conversion2/1
  Vref/1 -> Rate Transition3/1
  Switch2/1 -> Mux2/1, Mux/2, Cast To Boolean/1, Logical Operator/1
  [Iac_abs] -> Bus Creator/2  "Iac_abc"
  AbsV/1 -> Prod1/1
  PLL/1 -> Terminator/1
  Rate Transition5/1 -> AbsI/1, [i_L]
  Bus Creator/1 -> Sig/1
  Prod1/1 -> PR2/1(Iref), [Iref]
  Vac/1 -> Rate Transition/1
  PWM Generator (DC-DC)/1 -> Switch2/3
  Cast To Boolean/1 -> [u_PWM]
  RT/1 -> [u_obs], Switch2/1
  [Iref_obs] -> Bus Creator/1  "Iref_obs"
  [mcp_full_bridge_o] -> RT/1
  Vdc/1 -> Rate Transition4/1
  Mux2/1 -> Switch1/3
  [u_obs] -> Bus Creator1/1  "u_obs"
  Rate Transition4/1 -> [V_o], Speed Regulator2/2(Vmeas)
  Switch1/1 -> On Delay/1
  Rate Transition3/1 -> Speed Regulator2/1(Vref)
  [D] -> Bus Creator/3  "D"
  Trigonometric Function7/1 -> [Iref_obs], Rate Transition2/1, AbsV/1
  AbsI/1 -> [Iac_abs], PR2/2(Iac)
  Bus Creator1/1 -> u_swt/1
  Rate Transition/1 -> to-pu/1, [V_in]
  to-pu/1 -> PLL/1
  Saturation/1 -> [D], PWM Generator (DC-DC)/1
  PLL/2 -> Trigonometric Function7/1, [theta_pll]
  Data Type Conversion2/1 -> g1_g2/1
  Rate Transition2/1 -> Switch1/2
  Speed Regulator2/1(Out) -> Prod1/2
  Iac/1 -> Rate Transition5/1, [Iac]
  Mux/1 -> Switch1/1

== system PV_MEV/EV System1/Subsystem ==

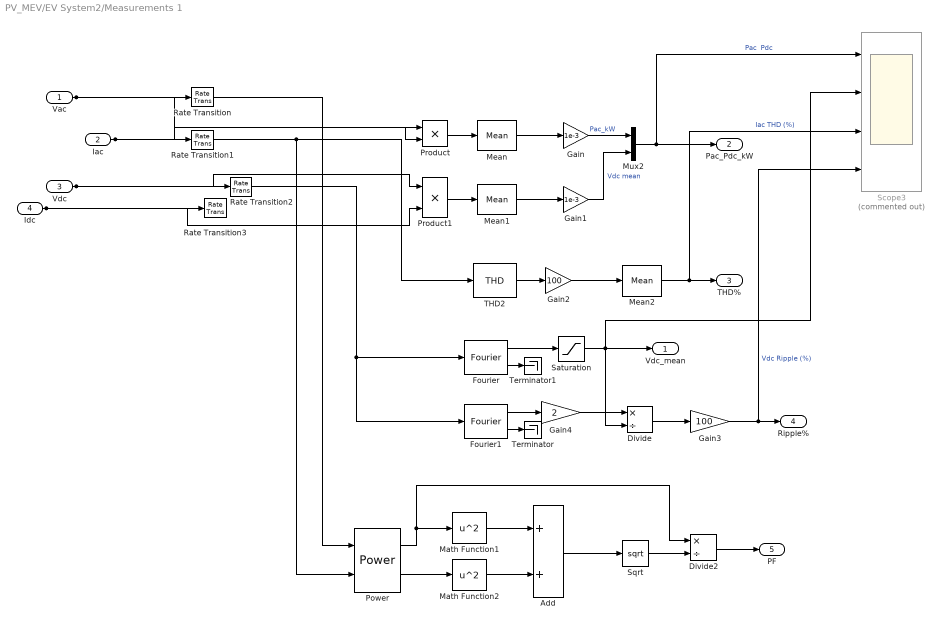
== system PV_MEV/EV System2/Measurements 1 ==
  Vac : Inport
  Iac : Inport  Port=2
  Vdc : Inport  Port=3
  Idc : Inport  Port=4
  Add : Sum
  Divide : Product  Inputs=*/
  Divide2 : Product  Inputs=*/
  Fourier : spsFourierLib/Fourier  Freq=Fnom  n=0  InInit=[0, 0]  Ts=Ts_Control
  Fourier1 : spsFourierLib/Fourier  Freq=Fnom  n=2  InInit=[0, 0]  Ts=Ts_Control
  Gain : Gain  Gain=1e-3
  Gain1 : Gain  Gain=1e-3
  Gain2 : Gain  Gain=100
  Gain3 : Gain  Gain=100
  Gain4 : Gain  Gain=2
  Math Function1 : Math  Operator=square
  Math Function2 : Math  Operator=square
  Mean : spsMeanLib/Mean  Freq=Fnom  Vinit=0  Ts=Ts_Power
  Mean1 : spsMeanLib/Mean  Freq=Fnom  Vinit=0  Ts=Ts_Power
  Mean2 : spsMeanLib/Mean  Freq=Fnom  Vinit=0  Ts=Ts_Control
  Mux2 : Mux  Inputs=2
  Power : spsPowerLib/Power  Freq=Fnom  Vinit=[1, 0]  Iinit=[1, 0]  Ts=Ts_Control
  Product : Product
  Product1 : Product
  Rate Transition{,1..3} (4 alike) : RateTransition  OutPortSampleTime=Ts_Control
  Saturation : Saturate  UpperLimit=inf  LowerLimit=eps
  Scope3 : Scope  Commented=on  NumInputPorts=4
      settings: DataLoggingSaveFormat=Array
  Sqrt : Sqrt
  THD2 : spsTHDLib/THD  Freq=Fnom  Ts=Ts_Control
  Terminator : Terminator
  Terminator1 : Terminator
  Vdc_mean : Outport
  Pac_Pdc_kW : Outport  Port=2
  THD% : Outport  Port=3
  Ripple% : Outport  Port=4
  PF : Outport  Port=5
  wires:
  Gain1/1 -> Mux2/2  "Vdc mean"
  Product1/1 -> Mean1/1
  Mean/1 -> Gain/1
  Product/1 -> Mean/1
  Gain/1 -> Mux2/1  "Pac_kW"
  THD2/1 -> Gain2/1
  Mean1/1 -> Gain1/1
  Iac/1 -> Rate Transition1/1, Product/2
  Mux2/1 -> Scope3/1, Pac_Pdc_kW/1  "Pac  Pdc"
  Gain2/1 -> Mean2/1
  Mean2/1 -> Scope3/3, THD%/1  "Iac THD (%)"
  Fourier/2 -> Terminator1/1
  Fourier/1 -> Saturation/1
  Saturation/1 -> Scope3/2, Vdc_mean/1, Divide/2
  Divide/1 -> Gain3/1
  Fourier1/1 -> Gain4/1
  Gain4/1 -> Divide/1
  Fourier1/2 -> Terminator/1
  Gain3/1 -> Scope3/4, Ripple%/1  "Vdc Ripple (%)"
  Power/1 -> Math Function1/1, Divide2/1
  Power/2 -> Math Function2/1
  Math Function1/1 -> Add/1
  Math Function2/1 -> Add/2
  Add/1 -> Sqrt/1
  Sqrt/1 -> Divide2/2
  Divide2/1 -> PF/1
  Rate Transition1/1 -> Power/2, THD2/1
  Vdc/1 -> Rate Transition2/1, Product1/1
  Idc/1 -> Rate Transition3/1, Product1/2
  Rate Transition/1 -> Power/1
  Vac/1 -> Rate Transition/1, Product/1
  Rate Transition2/1 -> Fourier/1, Fourier1/1

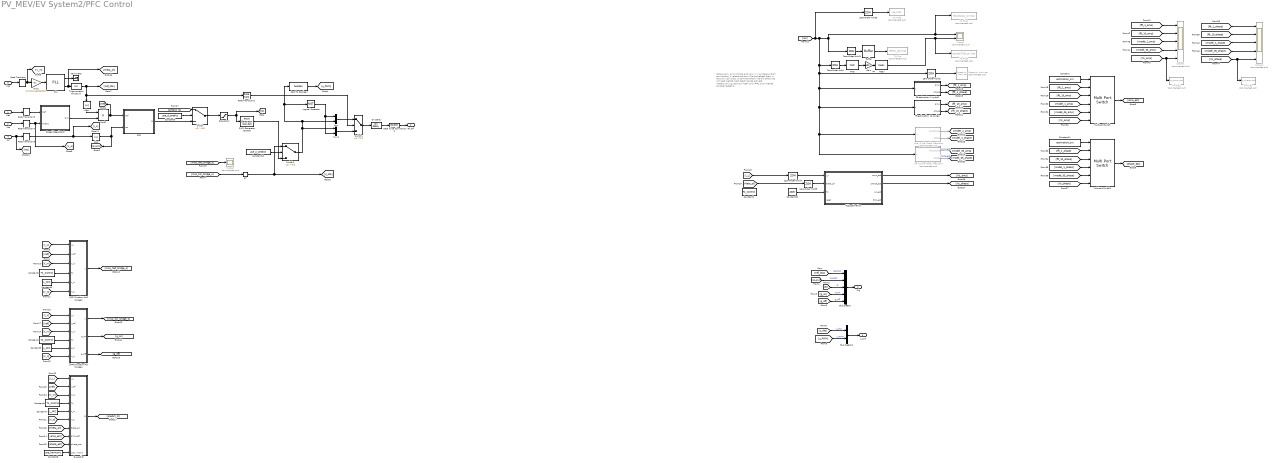
== system PV_MEV/EV System2/PFC Control ==
  note: Make sure
      | 1. onnxruntime and onnx in your base python enviroment.
      | 2. reload the onnx file and refresh them in the onnx call block.
      | or comment them like this
      | otherwise will lead matlab crash
      |
      | (bash)
      | conda activate matlab_onnx_py310
      | pip install onnx==1.14.0
      |
      | (matlab console)
      | target = "/home/changhong/anaconda3/envs/matlab_onnx_py310/bin/python";
      | pe = pyenv
      | pyenv("Version", target)
  Vref : Inport
  Vdc : Inport  Port=2
  Vac : Inport  Port=3
  Iac : Inport  Port=4
  AbsI : Abs  SaturateOnIntegerOverflow=off
  AbsV : Abs  SaturateOnIntegerOverflow=off
  Buffer : Buffer  N=80  V=79  OutputFrames=off
  Bus Creator : BusCreator  Inputs=5
  Bus Creator1 : BusCreator  Inputs=2
  Cast To Boolean : DataTypeConversion  OutDataTypeStr=boolean  SaturateOnIntegerOverflow=off  RndMeth=Floor
  Constant : Constant  Value=estimation_src
  Constant{1..2,4,6} (4 alike) : Constant  Value=Ts_Control
  Constant10 : Constant  Value=use_p_predict
  Constant11 : Constant  Value=estimation_src
  Constant12 : Constant  Value=4000
  Constant3 : Constant  Value=L_PFC
  Constant5 : Constant  Value=L_PFC
  Constant7 : Constant  Value=L_PFC
  Constant8 : Constant  Value=use_harmonic
  Constant9 : Constant  Value=use_d_predict
  D_predict : MATLAB Function  TreatAsAtomicUnit=on
  Data Type Conversion2 : DataTypeConversion  OutDataTypeStr=double  SaturateOnIntegerOverflow=off  RndMeth=Floor
  Gain : Gain  Gain=100
  Half Cycle Model Prediction : Subsystem  Commented=on
  Logical Operator : Logic  Operator=NOT  AllPortsSameDT=off  OutDataTypeStr=float('double')
  MCP Function Half bridge1 : MATLAB Function  TreatAsAtomicUnit=on
  Mean : spsMeanLib/Mean  Freq=50  Vinit=0  Ts=1/4000
  Multiport Switch : MultiPortSwitch  Inputs=5  SaturateOnIntegerOverflow=off  InputSameDT=off
  Multiport Switch1 : MultiPortSwitch  Inputs=5  SaturateOnIntegerOverflow=off  InputSameDT=off
  Mux : Mux  Inputs=2
  Mux2 : Mux  Inputs=2
  On Delay : spsOnDelayLib/On Delay  DelayType=On delay  delay=DT_PFC  ic=0  Ts=Ts_Power
  One  Cycle Model Prediction : Subsystem  Commented=on
  PLL : spsPLLLib/PLL  Fmin=0.9*Fnom  Par_Init=[0, Fnom]  ParK=[180, 3200, 1]  TcD=1e-4  MaxRateChangeFreq=12  FilterCutOffFreq=25  Ts=Ts_Control  AGC=on
  PR2 : Subsystem  mask(Current Regulator (Pr)){Kp=Kp_I, Kr=Kr_I, Fr=Fr_I}
      mask prompts: Kp "Proportional gain"; Kr "Resonant gain"; Fr "Resonant frequency (Hz)"
      mask help: This block implements a currentregulator using a PR controller.
      mask Display: disp('Current Regulator\n PR');
  PWM Generator (DC-DC) : spsPWMGeneratorDCDCLib/PWM Generator (DC-DC)  Fsw=Fsw  Ts=Ts_Power
  Prod1 : Product
  RLS_estimation : MATLAB Function  TreatAsAtomicUnit=on
  RT : RateTransition  OutPortSampleTime=5e-08
  Rate Transition{,3..5} (4 alike) : RateTransition  OutPortSampleTime=Ts_Control
  Rate Transition2 : RateTransition  OutPortSampleTime=Ts_Power
  Saturation : Saturate  UpperLimit=1  LowerLimit=0
  Scope : Scope  Commented=on  NumInputPorts=2
      settings: ActiveDisplayYMinimum=-211.219  ActiveDisplayYMaximum=223.7073  DataLoggingVariableName=ScopeData4  DataLoggingSaveFormat=Array
  Scope1 : Scope  Commented=on  NumInputPorts=5
      settings: ActiveDisplayYMinimum=-19.4864  ActiveDisplayYMaximum=175.3777  DataLoggingVariableName=ScopeData5  DataLoggingSaveFormat=Array
  Scope2 : Scope  Commented=on
      settings: DataLoggingVariableName=ScopeData9  DataLoggingSaveFormat=Array
  Scope3 : Scope  Commented=on  NumInputPorts=5
      settings: ActiveDisplayYMinimum=-3.927  ActiveDisplayYMaximum=3.927  DataLoggingVariableName=ScopeData6  DataLoggingSaveFormat=Array
  Spectrum Analyzer : SpectrumAnalyzer  Commented=on  WindowPosition=[-2559.000000,62.000000,1707.000000,996.000000,]  ScopeFrameLocation=window  SampleRateSource=Property  SampleRate=8000  PlotAsTwoSidedSpectrum=off  WindowInvariantSamplesPerUpdate=on  FrequencySpan=Start and stop frequencies  StartFrequency=0  StopFrequency=2000  YLimits=[-21.57310057,75.63654601]  ColorLimits=[-42.4528 59.157]
  Speed Regulator2 : Subsystem  DialogController=POWERSYS.PowerSysDialog  mask(Voltage Regulator){Kp=Kp_V, Ki=Ki_V, Limit_wreg=Limit_V, Init=0, Ts=Ts_Control}
      mask prompts: Kp "Proportional gain (Kp):"; Ki "Integral gain (Ki):"; Limit_wreg "Output limits"; Init "Output initial value:"; Ts "Sample time:"
      mask help: This block implements a voltage regulator using an ant-windup PI controller.
      mask Display: disp('Voltage\nRegulator');
  Switch : Switch  Criteria=u2 > Threshold  Threshold=0.5  SaturateOnIntegerOverflow=off  InputSameDT=off
  Switch1 : Switch  SaturateOnIntegerOverflow=off  InputSameDT=off
  Switch2 : Switch  Criteria=u2 > Threshold  Threshold=0.5  SaturateOnIntegerOverflow=off  InputSameDT=off
  THD : spsTHDLib/THD  Freq=50  Ts=1/4000
  Terminator : Terminator
  To File : ToFile  Commented=on  Filename=MPCC_IAC.mat  SaveFormat=Timeseries
  To File1 : ToFile  Commented=on  Filename=rls_phase.mat  SaveFormat=Timeseries
  To File2 : ToFile  Commented=on  Filename=rls_amp.mat  SaveFormat=Timeseries
  To File3 : ToFile  Commented=on  Filename=Iac.mat  SaveFormat=Timeseries
  To File4 : ToFile  Commented=on  Filename=results/Iac_ori.mat  SaveFormat=Timeseries
  To File5 : ToFile  Commented=on  Filename=results/THD_ori.mat  SaveFormat=Timeseries
  Trigonometric Function7 : Trigonometry
  UMPC Function Full bridge1 : MATLAB Function  TreatAsAtomicUnit=on
  Zero-Order Hold{,1,3..5} (5 alike) : ZeroOrderHold  SampleTime=1/4000
  Zero-Order Hold2 : ZeroOrderHold  SampleTime=1/8000
  fft estimation 1 cycle2 : Subsystem
  fft estimation 10 cycle2 : Subsystem
  to-pu : Gain  Gain=1/(Vnom_ac*sqrt(2))
  g1_g2 : Outport  PortDimensions=2
  Sig : Outport  Port=2
  u_swt : Outport  Port=3
  wires:
  Mux/1 -> Switch1/1
  Iac/1 -> [Iac], Rate Transition5/1
  Speed Regulator2/1(Out) -> Prod1/2
  Rate Transition2/1 -> Switch1/2
  Data Type Conversion2/1 -> g1_g2/1
  PLL/2 -> [theta_pll], Trigonometric Function7/1
  Saturation/1 -> PWM Generator (DC-DC)/1, [D]
  to-pu/1 -> PLL/1
  Rate Transition/1 -> [V_in], to-pu/1
  Bus Creator1/1 -> u_swt/1
  AbsI/1 -> PR2/2(Iac), [Iac_abs]
  Trigonometric Function7/1 -> AbsV/1, Rate Transition2/1, [Iref_obs]
  [D] -> Bus Creator/3  "D"
  Rate Transition3/1 -> Speed Regulator2/1(Vref)
  Switch1/1 -> On Delay/1
  Rate Transition4/1 -> Speed Regulator2/2(Vmeas), [V_o]
  [u_obs] -> Bus Creator1/1  "u_obs"
  Mux2/1 -> Switch1/3
  Vdc/1 -> Rate Transition4/1
  [mcp_full_bridge_o] -> RT/1
  [Iref_obs] -> Bus Creator/1  "Iref_obs"
  RT/1 -> Switch2/1, [u_obs]
  Cast To Boolean/1 -> [u_PWM]
  PWM Generator (DC-DC)/1 -> Switch2/3
  Vac/1 -> Rate Transition/1
  Prod1/1 -> [Iref], PR2/1(Iref)
  Bus Creator/1 -> Sig/1
  Rate Transition5/1 -> [i_L], AbsI/1
  PLL/1 -> Terminator/1
  AbsV/1 -> Prod1/1
  [Iac_abs] -> Bus Creator/2  "Iac_abc"
  Switch2/1 -> Logical Operator/1, Cast To Boolean/1, Mux/2, Mux2/1
  Vref/1 -> Rate Transition3/1
  On Delay/1 -> Data Type Conversion2/1
  [u_PWM] -> Bus Creator1/2  "u_PWM"
  [Iac] -> Zero-Order Hold3/1, Half Cycle Model Prediction/1(u), One  Cycle Model Prediction/1(u), fft estimation 10 cycle2/1(u), fft estimation 1 cycle2/1(u), Zero-Order Hold2/1, Zero-Order Hold/1, Zero-Order Hold1/1, To File4/1, Scope/1  "Iac"
  Buffer/1 -> To File/1
  Gain/1 -> Mean/1
  Zero-Order Hold/1 -> THD/1
  Mean/1 -> To File5/1, Scope/2
  Zero-Order Hold2/1 -> Spectrum Analyzer/1
  THD/1 -> Gain/1
  Zero-Order Hold1/1 -> Buffer/1
  [i_L] -> MCP Function Half bridge1/1(i_L)
  [Iref] -> MCP Function Half bridge1/2(i_ref)
  [V_in] -> MCP Function Half bridge1/3(V_in)
  Constant2/1 -> MCP Function Half bridge1/4(Ts)
  Constant3/1 -> MCP Function Half bridge1/5(L_in)
  [V_o] -> MCP Function Half bridge1/6(V_o)
  MCP Function Half bridge1/1(y) -> [mcp_half_bridge_o]
  [i_L] -> UMPC Function Full bridge1/1(i_L)
  [Iref] -> UMPC Function Full bridge1/2(i_ref)
  [V_in] -> UMPC Function Full bridge1/3(V_in)
  Constant4/1 -> UMPC Function Full bridge1/4(Ts)
  Constant5/1 -> UMPC Function Full bridge1/5(L_in)
  [V_o] -> UMPC Function Full bridge1/6(V_o)
  UMPC Function Full bridge1/1(y) -> [mcp_full_bridge_o]
  UMPC Function Full bridge1/2(g_on) -> [g_on]
  UMPC Function Full bridge1/3(g_off) -> [g_off]
  [g_on] -> Bus Creator/4  "g_on"
  [g_off] -> Bus Creator/5  "g_off"
  [theta_pll] -> Zero-Order Hold5/1
  [i_L] -> D_predict/1(i_L)
  [Iref] -> D_predict/2(i_ref)
  [V_in] -> D_predict/3(V_in)
  Constant6/1 -> D_predict/4(Ts)
  Constant7/1 -> D_predict/5(L_in)
  [V_o] -> D_predict/6(V_o)
  [amp_est] -> D_predict/8(amp_est)
  [phase_est] -> D_predict/9(phase_est)
  Constant8/1 -> D_predict/10(use_harmonic)
  [theta_pll] -> D_predict/7(theta_pll)
  D_predict/1(D) -> [predict_D]
  [mcp_half_bridge_o] -> Scope2/1
  Constant9/1 -> Switch/2
  [predict_D] -> Switch/1
  PR2/1(D) -> Switch/3
  Switch/1 -> Saturation/1
  Constant10/1 -> Switch2/2
  Logical Operator/1 -> Mux2/2, Mux/1
  Constant/1 -> Multiport Switch/1
  fft estimation 1 cycle2/1(amp) -> [fft_1_amp]
  fft estimation 1 cycle2/2(phase) -> [fft_1_phase]
  fft estimation 10 cycle2/1(amp) -> [fft_10_amp]
  fft estimation 10 cycle2/2(phase) -> [fft_10_phase]
  One  Cycle Model Prediction/1(amplitude) -> [model_1_amp]
  One  Cycle Model Prediction/2(phase) -> [model_1_phase]
  Half Cycle Model Prediction/1(amplitude) -> [model_05_amp]  "amp_est"
  Half Cycle Model Prediction/2(phase) -> [model_05_phase]  "hase_est"
  Multiport Switch/1 -> [amp_est]
  RLS_estimation/1(amp_est) -> [rls_amp]
  RLS_estimation/2(phase_est) -> [rls_phase]
  [fft_1_amp] -> Multiport Switch/2
  [fft_10_amp] -> Multiport Switch/3
  [model_1_amp] -> Multiport Switch/4
  [model_05_amp] -> Multiport Switch/5
  [rls_amp] -> Multiport Switch/6
  [rls_phase] -> Multiport Switch1/6
  [model_05_phase] -> Multiport Switch1/5
  [model_1_phase] -> Multiport Switch1/4
  [fft_10_phase] -> Multiport Switch1/3
  [fft_1_phase] -> Multiport Switch1/2
  Multiport Switch1/1 -> [phase_est]
  Constant11/1 -> Multiport Switch1/1
  [fft_1_amp] -> Scope1/1
  [fft_10_amp] -> Scope1/2
  [model_1_amp] -> Scope1/3
  [model_05_amp] -> Scope1/4
  [rls_amp] -> To File2/1, Scope1/5
  [fft_1_phase] -> Scope3/1
  [fft_10_phase] -> Scope3/2
  [model_1_phase] -> Scope3/3
  [model_05_phase] -> Scope3/4
  [rls_phase] -> To File1/1, Scope3/5
  Zero-Order Hold3/1 -> To File3/1
  [i_L] -> Zero-Order Hold4/1
  Constant12/1 -> RLS_estimation/3(Ts)
  Zero-Order Hold4/1 -> RLS_estimation/1(i_L)
  Zero-Order Hold5/1 -> RLS_estimation/2(theta_pll)

== system PV_MEV/EV System2/Subsystem ==

== system PV_MEV/PV System/DC AC Inverter ==
  note: 500V
      | 3-level VSC
  3-Level Bridge : spsThreeLevelBridgeLib/Three-Level Bridge  Arms=3  SnubberResistance=1e6  SbubberCapacitance=inf  Device=IGBT / Diodes  Ron=0.2e-3  ForwardVoltages="[  0  0 ]"  Measurements=None
      settings: AttributesFormatString=\n
  Deblock Converters : Step  Time=0.05  SampleTime=0
  Product1 : Product  RndMeth=Zero
  VSC Control : Subsystem  mask(VSC Main Controller){nom=[ 100e3  Fnom ], Vnom=[ 25e3 Vnom_ac ], Vnom_dc=500, RLxfo=[0.002  0.06 ], RLchoke=[2e-3  250e-6  ], K_VDCreg=[7  800], K_Ireg=[0.3 20], Ts=Ts_Control}
      mask prompts: nom "Nominal power and frequency [ Pnom(VA)  Fnom(Hz) ]:"; Vnom "Nominal primary and secondary voltages (Vrms LL) [ Vnom_prim   Vnom_sec ]:"; Vnom_dc "Nominal DC bus voltage (V):"; RLxfo "Total transformer leakage impedance (pu/Pnom) [ Rxfo  Lxf ]"; RLchoke "Choke impedance [ R(ohm) L(H) ]"; K_VDCreg "VDC regultator gains [ Kp  Ki ]:"; K_Ireg "Current regulator gains [ Kp  Ki ]:"; Ts "Sample time"
      mask init:
      | Pnom=nom(1);
      | Fnom=nom(2);
      | Vnom_prim=Vnom(1);
      | Vnom_sec=Vnom(2);
      | Zbase=Vnom_sec^2/Pnom;
      | Rtot_pu=RLxfo(1) + RLchoke(1)/Zbase;
      | Ltot_pu=RLxfo(2) + RLchoke(2)/(Zbase/(2*pi*Fnom));
      | Kp_VDCreg=K_VDCreg(1);
      | Ki_VDCreg=K_VDCreg(2);
      | Kp_Ireg=K_Ireg(1);
      | Ki_Ireg=K_Ireg(2);
      | Vdc_ref=Vnom_dc;
      | % Used to determine initial value of Boost Control (MPPT)
      | assignin('base','Vdc_ref_Inv',Vdc_ref);
  DC + IN : PMIOPort  Side=Left
  DC Mid IN : PMIOPort  Port=2  Side=Left
  DC - IN : PMIOPort  Port=3  Side=Left
  A : PMIOPort  Port=4  Side=Right
  B : PMIOPort  Port=5  Side=Right
  C : PMIOPort  Port=6  Side=Right
  wires:
  [Iabc_B1] -> VSC Control/2(Iabc_prim)
  VSC Control/1(Pulses) -> Product1/2
  [Vdc] -> VSC Control/3(Vdc_mes)
  [Vabc_B1] -> VSC Control/1(Vabc_prim)
  Product1/1 -> 3-Level Bridge/1
  Deblock Converters/1 -> Product1/1
  connections:
  DC + IN/RConn1 -- 3-Level Bridge/RConn1
  DC Mid IN/RConn1 -- 3-Level Bridge/RConn2
  DC - IN/RConn1 -- 3-Level Bridge/RConn3
  3-Level Bridge/LConn1 -- A/RConn1
  3-Level Bridge/LConn2 -- B/RConn1
  3-Level Bridge/LConn3 -- C/RConn1
